simulink model "CAVE_MachE_speedTrack0202"  (R2019b)
settings: configuration reference "ConfigSetDesktopFixedStep" (kept outside this file)
PreLoadFcn:
  | VSS_BICYCLE=Simulink.Variant('Dual=0');
  | VSS_DUAL=Simulink.Variant('Dual=1');
  | Dual=1;
  | load('DriveCycle2.mat')
PostLoadFcn:
  | if any(exist('dsrtsu_mdlpostloadfcn', 'file') ~= 0), dsrtsu_mdlpostloadfcn('Execute', bdroot); end
InitFcn:
  | , if any(exist('dsmpb_private', 'file') ~= 0), dsmpb_private('dsmpb_mdlclblib', 'Init', bdroot); end,
  | load('DriveCycle2.mat')
model workspace (MAT data in the model file):
  Gas = 0.383333333333
values from neighbouring files (symbols this model uses):
  CoastDown =     [Run_Simulink.mat]
  limitedMCT =     [Run_Simulink.mat]
  MCT =     [Run_Simulink.mat]
  pMCT =     [Run_Simulink.mat]
  Ref_speed = [13 13.007895099 13.015778396 13.023649891 13.031509584 13.039357475 13.047193564 13.055017851 13.062830336 13.070631019 13.0784199 13.086196979 ... (2669 elements, 2669x1)]    [Ref_speed_and_time.mat]
  Ref_time = [0 0.01 0.02 0.03 0.04 0.05 0.06 0.07 0.08 0.09 0.1 0.11 ... (2669 elements, 2669x1)]    [Ref_speed_and_time.mat]
  US06 =     [Run_Simulink.mat]
undefined symbols (not defined in the file or in its folder): AccelCmd, ActTqLF_Nm_, ActTqLR_Nm_, ActTqRF_Nm_, ActTqRR_Nm_, BattChargeLimitMaxPwr, BattChargeLimitSocBpts, BattChargeLimitTbl, BattChrgCapcty, BattDischargeLimitSocBpts, BattDischargeLimitTbl, BattDischargeMaxPwr, BattNumCellsParallel, BattNumCellsSeries, BattOpenVoltCapBpts, BattOpenVoltTbl, BattResistSocBpts, BattResistTbl, BattResistTempBpts, BrakeMaxPrs, BrakeMaxTrq, ChassisDistCg2FrontAxle, ChassisDistCg2RearAxle, ChassisVehMass, CltchCmd, DecelCmd, DiffRatio, DiscIntNeverNeededParam, EnvGravCnst, EnvPrs, EnvTemp, FuelSpecificGrav, GearCmd, h, InitStates, lgSw, MtrEffSpdBpts, MtrEffTbl, MtrEffTrqBpts, MtrPwrMax, MtrTrqMax, Ref_Spd0229, Ref_Time0229, SteeringCmd, SupvsryCtrlRegenBrkCutOffTbl, SupvsryCtrlRegenSpdBpts, TestScnrioCycleNum, VEH
libraries: VSIGenLib x67, simulink x57, etargetslib x38, dsmpblib x28, vehdynlibtire x12, autolibshared x9, vehdynlibsuspension x7, vehdynlibtirecommon x7, autolibutils x5, CarMaker4SL x4, VsrLibWheel x4, autolibpowerinfoutils x3
(part 5 of 14)

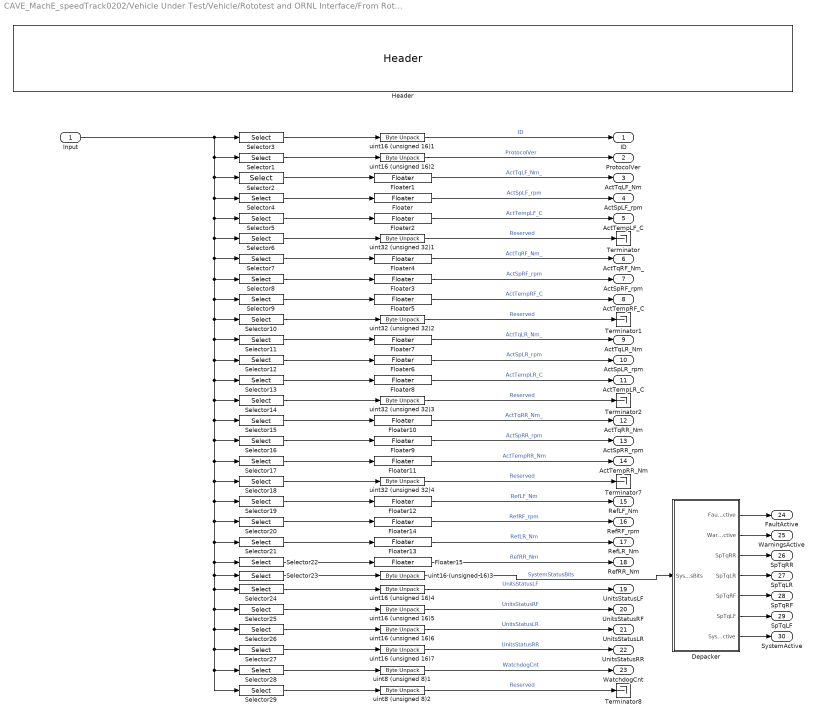
== system CAVE_MachE_speedTrack0202/Vehicle Under Test/Vehicle/Rototest and ORNL Interface/From Rototest/RotoTestEthRX ==
  Input : Inport
  Depacker : Subsystem
  Floater{,1..15} (16 alike) : VSIGenLib/Floater  SystemSampleTime=-1  Latency=0  AutoFrameSizeCalculation=off
  Header : VSIGenLib/Header  not=''
  Selector1 : Selector  IndexMode=Zero-based  InputPortWidth=96  IndexOptions=Index vector (dialog)  Indices=[3 2]  OutputSizes=1
  Selector10 : Selector  IndexMode=Zero-based  InputPortWidth=96  IndexOptions=Index vector (dialog)  Indices=[35 34 33 32]  OutputSizes=1
  Selector11 : Selector  IndexMode=Zero-based  InputPortWidth=96  IndexOptions=Index vector (dialog)  Indices=[39 38 37 36]  OutputSizes=1
  Selector12 : Selector  IndexMode=Zero-based  InputPortWidth=96  IndexOptions=Index vector (dialog)  Indices=[43 42 41 40]  OutputSizes=1
  Selector13 : Selector  IndexMode=Zero-based  InputPortWidth=96  IndexOptions=Index vector (dialog)  Indices=[47 46 45 44]  OutputSizes=1
  Selector14 : Selector  IndexMode=Zero-based  InputPortWidth=96  IndexOptions=Index vector (dialog)  Indices=[51 50 49 48]  OutputSizes=1
  Selector15 : Selector  IndexMode=Zero-based  InputPortWidth=96  IndexOptions=Index vector (dialog)  Indices=[55 54 53 52]  OutputSizes=1
  Selector16 : Selector  IndexMode=Zero-based  InputPortWidth=96  IndexOptions=Index vector (dialog)  Indices=[59 58 57 56]  OutputSizes=1
  Selector17 : Selector  IndexMode=Zero-based  InputPortWidth=96  IndexOptions=Index vector (dialog)  Indices=[63 62 61 60]  OutputSizes=1
  Selector18 : Selector  IndexMode=Zero-based  InputPortWidth=96  IndexOptions=Index vector (dialog)  Indices=[67 66 65 64]  OutputSizes=1
  Selector19 : Selector  IndexMode=Zero-based  InputPortWidth=96  IndexOptions=Index vector (dialog)  Indices=[71 70 69 68]  OutputSizes=1
  Selector2 : Selector  IndexMode=Zero-based  InputPortWidth=96  IndexOptions=Index vector (dialog)  Indices=[7 6 5 4]  OutputSizes=1
  Selector20 : Selector  IndexMode=Zero-based  InputPortWidth=96  IndexOptions=Index vector (dialog)  Indices=[75 74 73 72]  OutputSizes=1
  Selector21 : Selector  IndexMode=Zero-based  InputPortWidth=96  IndexOptions=Index vector (dialog)  Indices=[79 78 77 76]  OutputSizes=1
  Selector22 : Selector  IndexMode=Zero-based  InputPortWidth=96  IndexOptions=Index vector (dialog)  Indices=[83 82 81 80]  OutputSizes=1
  Selector23 : Selector  IndexMode=Zero-based  InputPortWidth=96  IndexOptions=Index vector (dialog)  Indices=[85 84]  OutputSizes=1
  Selector24 : Selector  IndexMode=Zero-based  InputPortWidth=96  IndexOptions=Index vector (dialog)  Indices=[87 86]  OutputSizes=1
  Selector25 : Selector  IndexMode=Zero-based  InputPortWidth=96  IndexOptions=Index vector (dialog)  Indices=[89 88]  OutputSizes=1
  Selector26 : Selector  IndexMode=Zero-based  InputPortWidth=96  IndexOptions=Index vector (dialog)  Indices=[91 90]  OutputSizes=1
  Selector27 : Selector  IndexMode=Zero-based  InputPortWidth=96  IndexOptions=Index vector (dialog)  Indices=[93 92]  OutputSizes=1
  Selector28 : Selector  IndexMode=Zero-based  InputPortWidth=96  IndexOptions=Index vector (dialog)  Indices=[94]  OutputSizes=1
  Selector29 : Selector  IndexMode=Zero-based  InputPortWidth=96  IndexOptions=Index vector (dialog)  Indices=[95]  OutputSizes=1
  Selector3 : Selector  IndexMode=Zero-based  InputPortWidth=96  IndexOptions=Index vector (dialog)  Indices=[1 0]  OutputSizes=1
  Selector4 : Selector  IndexMode=Zero-based  InputPortWidth=96  IndexOptions=Index vector (dialog)  Indices=[11 10 9 8]  OutputSizes=1
  Selector5 : Selector  IndexMode=Zero-based  InputPortWidth=96  IndexOptions=Index vector (dialog)  Indices=[15 14 13 12]  OutputSizes=1
  Selector6 : Selector  IndexMode=Zero-based  InputPortWidth=96  IndexOptions=Index vector (dialog)  Indices=[19 18 17 16]  OutputSizes=1
  Selector7 : Selector  IndexMode=Zero-based  InputPortWidth=96  IndexOptions=Index vector (dialog)  Indices=[23 22 21 20]  OutputSizes=1
  Selector8 : Selector  IndexMode=Zero-based  InputPortWidth=96  IndexOptions=Index vector (dialog)  Indices=[27 26 25 24]  OutputSizes=1
  Selector9 : Selector  IndexMode=Zero-based  InputPortWidth=96  IndexOptions=Index vector (dialog)  Indices=[31 30 29 28]  OutputSizes=1
  Terminator{,1..2,7..8} (5 alike) : Terminator
  uint16 (unsigned 16){1..7} (7 alike) : etargetslib/Byte Unpack  dimensions={[1]}  datatypes={'uint16'}  byteAlign=1
      settings: SourceProductName=MATLAB Coder
  uint32 (unsigned 32){1..4} (4 alike) : etargetslib/Byte Unpack  dimensions={[1]}  datatypes={'uint32'}  byteAlign=1
      settings: SourceProductName=MATLAB Coder
  uint8 (unsigned 8)1 : etargetslib/Byte Unpack  dimensions={[1]}  datatypes={'uint8'}  byteAlign=1
      settings: SourceProductName=MATLAB Coder
  uint8 (unsigned 8)2 : etargetslib/Byte Unpack  dimensions={[1]}  datatypes={'uint8'}  byteAlign=1
      settings: SourceProductName=MATLAB Coder
  ID : Outport
  ProtocolVer : Outport  Port=2
  ActTqLF_Nm : Outport  Port=3
  ActSpLF_rpm : Outport  Port=4
  ActTempLF_C : Outport  Port=5
  ActTqRF_Nm_ : Outport  Port=6
  ActSpRF_rpm : Outport  Port=7
  ActTempRF_C : Outport  Port=8
  ActTqLR_Nm : Outport  Port=9
  ActSpLR_rpm : Outport  Port=10
  ActTempLR_C : Outport  Port=11
  ActTqRR_Nm : Outport  Port=12
  ActSpRR_rpm : Outport  Port=13
  ActTempRR_Nm : Outport  Port=14
  RefLF_Nm : Outport  Port=15
  RefRF_rpm : Outport  Port=16
  RefLR_Nm : Outport  Port=17
  RefRR_Nm : Outport  Port=18
  UnitsStatusLF : Outport  Port=19
  UnitsStatusRF : Outport  Port=20
  UnitsStatusLR : Outport  Port=21
  UnitsStatusRR : Outport  Port=22
  WatchdogCnt : Outport  Port=23
  FaultActive : Outport  Port=24
  WarningsActive : Outport  Port=25
  SpTqRR : Outport  Port=26
  SpTqLR : Outport  Port=27
  SpTqRF : Outport  Port=28
  SpTqLF : Outport  Port=29
  SystemActive : Outport  Port=30
  wires:
  Depacker/7(SystemActive) -> SystemActive/1
  Depacker/5(SpTqRF) -> SpTqRF/1
  Depacker/1(FaultActive) -> FaultActive/1
  Depacker/2(WarningsActive) -> WarningsActive/1
  Depacker/3(SpTqRR) -> SpTqRR/1
  Depacker/4(SpTqLR) -> SpTqLR/1
  Depacker/6(SpTqLF) -> SpTqLF/1
  Floater5/1 -> ActTempRF_C/1  "ActTempRF_C"
  uint32 (unsigned 32)2/1 -> Terminator1/1  "Reserved"
  Floater/1 -> ActSpLF_rpm/1  "ActSpLF_rpm"
  uint32 (unsigned 32)1/1 -> Terminator/1  "Reserved"
  uint16 (unsigned 16)1/1 -> ID/1  "ID"
  Floater15/1 -> RefRR_Nm/1  "RefRR_Nm"
  uint8 (unsigned 8)1/1 -> WatchdogCnt/1  "WatchdogCnt"
  Floater14/1 -> RefRF_rpm/1  "RefRF_rpm"
  uint16 (unsigned 16)5/1 -> UnitsStatusRF/1  "UnitsStatusRF"
  uint32 (unsigned 32)3/1 -> Terminator2/1  "Reserved"
  Floater9/1 -> ActSpRR_rpm/1  "ActSpRR_rpm"
  Floater1/1 -> ActTqLF_Nm/1  "ActTqLF_Nm_"
  Floater2/1 -> ActTempLF_C/1  "ActTempLF_C"
  Floater12/1 -> RefLF_Nm/1  "RefLF_Nm"
  Floater7/1 -> ActTqLR_Nm/1  "ActTqLR_Nm_"
  uint16 (unsigned 16)2/1 -> ProtocolVer/1  "ProtocolVer"
  Selector24/1 -> uint16 (unsigned 16)4/1
  Selector7/1 -> Floater4/1
  Selector8/1 -> Floater3/1
  uint16 (unsigned 16)7/1 -> UnitsStatusRR/1  "UnitsStatusRR"
  Selector22/1 -> Floater15/1
  Selector18/1 -> uint32 (unsigned 32)4/1
  Selector12/1 -> Floater6/1
  Selector23/1 -> uint16 (unsigned 16)3/1
  uint16 (unsigned 16)6/1 -> UnitsStatusLR/1  "UnitsStatusLR"
  Selector17/1 -> Floater11/1
  uint16 (unsigned 16)4/1 -> UnitsStatusLF/1  "UnitsStatusLF"
  Selector27/1 -> uint16 (unsigned 16)7/1
  Floater13/1 -> RefLR_Nm/1  "RefLR_Nm"
  Selector14/1 -> uint32 (unsigned 32)3/1
  Selector2/1 -> Floater1/1
  Selector13/1 -> Floater8/1
  Selector26/1 -> uint16 (unsigned 16)6/1
  Selector6/1 -> uint32 (unsigned 32)1/1
  uint16 (unsigned 16)3/1 -> Depacker/1(SysStsBits)  "SystemStatusBits"
  uint32 (unsigned 32)4/1 -> Terminator7/1  "Reserved"
  Floater3/1 -> ActSpRF_rpm/1  "ActSpRF_rpm"
  Selector25/1 -> uint16 (unsigned 16)5/1
  Floater4/1 -> ActTqRF_Nm_/1  "ActTqRF_Nm_"
  uint8 (unsigned 8)2/1 -> Terminator8/1  "Reserved"
  Floater11/1 -> ActTempRR_Nm/1  "ActTempRR_Nm"
  Floater6/1 -> ActSpLR_rpm/1  "ActSpLR_rpm"
  Selector20/1 -> Floater14/1
  Selector9/1 -> Floater5/1
  Selector5/1 -> Floater2/1
  Selector15/1 -> Floater10/1
  Selector16/1 -> Floater9/1
  Floater8/1 -> ActTempLR_C/1  "ActTempLR_C"
  Selector3/1 -> uint16 (unsigned 16)1/1
  Selector28/1 -> uint8 (unsigned 8)1/1
  Selector29/1 -> uint8 (unsigned 8)2/1
  Selector21/1 -> Floater13/1
  Input/1 -> Selector7/1, Selector8/1, Selector9/1, Selector10/1, Selector11/1, Selector12/1, Selector13/1, Selector17/1, Selector18/1, Selector19/1, Selector20/1, Selector21/1, Selector22/1, Selector23/1, Selector25/1, Selector26/1, Selector27/1, Selector29/1, Selector28/1, Selector24/1, Selector16/1, Selector15/1, Selector14/1, Selector6/1, Selector5/1, Selector4/1, Selector2/1, Selector1/1, Selector3/1
  Selector19/1 -> Floater12/1
  Selector10/1 -> uint32 (unsigned 32)2/1
  Selector1/1 -> uint16 (unsigned 16)2/1
  Selector4/1 -> Floater/1
  Floater10/1 -> ActTqRR_Nm/1  "ActTqRR_Nm_"
  Selector11/1 -> Floater7/1

== system CAVE_MachE_speedTrack0202/Vehicle Under Test/Vehicle/Rototest and ORNL Interface/Get Wheel Spd Cmd Based on Wheel Dynamics/WheelSpdCmd ==
  In1 : Inport
  Bus Selector : BusSelector  OutputSignals=PT IF WFL rotv,PT IF WFR rotv,PT IF WRL rotv,PT IF WRR rotv
  Mux : Mux
  Out1 : Outport
  wires:
  Mux/1 -> Out1/1
  Bus Selector/1 -> Mux/1  "<PT IF WFL rotv>"
  Bus Selector/4 -> Mux/4  "<PT IF WRR rotv>"
  In1/1 -> Bus Selector/1
  Bus Selector/3 -> Mux/3  "<PT IF WRL rotv>"
  Bus Selector/2 -> Mux/2  "<PT IF WFR rotv>"

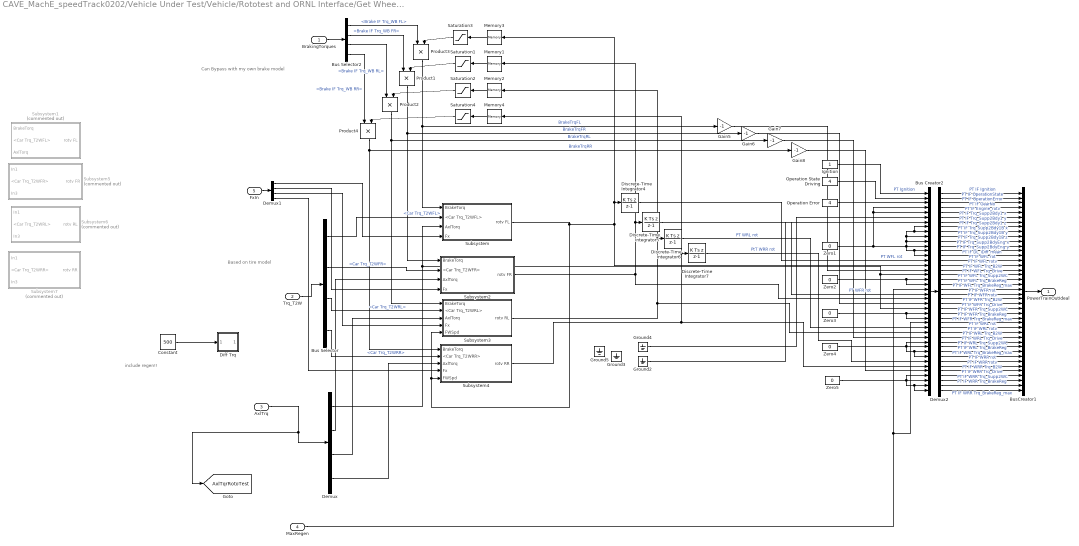
== system CAVE_MachE_speedTrack0202/Vehicle Under Test/Vehicle/Rototest and ORNL Interface/Get Wheel Spd Cmd Based on Wheel Dynamics/Whl Dynamics & Format CM Powertrain Signal ==
  note: include regen!!
  note: Based on tire model
  note: Can Bypass with my own brake model
  BrakingTorques : Inport
  Trq_T2W : Inport  Port=2
  AxlTrq : Inport  Port=3
  MaxRegen : Inport  Port=4
  FxIn : Inport  Port=5
  Bus Creator2 : BusCreator  Inputs=42
  Bus Selector : BusSelector  OutputSignals=Car Trq_T2WFL,Car Trq_T2WFR,Car Trq_T2WRL,Car Trq_T2WRR
  Bus Selector2 : BusSelector  OutputSignals=Brake IF Trq_WB FL,Brake IF Trq_WB FR,Brake IF Trq_WB RL,Brake IF Trq_WB RR
  BusCreator1 : BusCreator  Inputs=42
  Constant : Constant  Value=500
  Demux : Demux
  Demux1 : Demux
  Demux2 : Demux  Outputs=42
  Diff Trq : Subsystem
  Discrete-Time Integrator{4..7} (4 alike) : DiscreteIntegrator  IntegratorMethod=Integration: Backward Euler  SampleTime=-1  ICPrevOutput=DiscIntNeverNeededParam  ICPrevScaledInput=DiscIntNeverNeededParam
  Gain{5..8} (4 alike) : Gain  Gain=-1
  Ground{2..5} (4 alike) : Ground
  Ignition : Constant
  Memory{1..4} (4 alike) : Memory
  Operation Error : Constant  Value=4
  Operation State Driving : Constant  Value=4
  Product{1..4} (4 alike) : Product  RndMeth=Zero
  Saturation{1..4} (4 alike) : Saturate  UpperLimit=1  LowerLimit=-1
  Subsystem : Subsystem
  Subsystem1 : Subsystem  Commented=on
  Subsystem2 : Subsystem
  Subsystem3 : Subsystem
  Subsystem4 : Subsystem
  Subsystem5 : Subsystem  Commented=on
  Subsystem6 : Subsystem  Commented=on
  Subsystem7 : Subsystem  Commented=on
  Zero{1..5} (5 alike) : Constant  Value=0
  PowerTrainOutIdeal : Outport
  tag scope: AxlTqrRotoTest=global
  wires:
  Saturation4/1 -> Product4/2
  Memory4/1 -> Saturation4/1
  Bus Selector2/4 -> Product4/1  "<Brake IF Trq_WB RR>"
  Product4/1 -> Subsystem4/1(BrakeTorq), Gain8/1  "BrakeTrqRR"
  Saturation2/1 -> Product2/2
  Memory2/1 -> Saturation2/1
  Bus Selector2/3 -> Product2/1  "<Brake IF Trq_WB RL>"
  Product2/1 -> Subsystem3/1(BrakeTorq), Gain7/1  "BrakeTrqRL"
  Saturation1/1 -> Product1/2
  Memory1/1 -> Saturation1/1
  Bus Selector2/2 -> Product1/1  "<Brake IF Trq_WB FR>"
  Product1/1 -> Subsystem2/1(BrakeTorq), Gain6/1  "BrakeTrqFR"
  Memory3/1 -> Saturation3/1
  Saturation3/1 -> Product3/2
  Bus Selector2/1 -> Product3/1  "<Brake IF Trq_WB FL>"
  Product3/1 -> Subsystem/1(BrakeTorq), Gain5/1  "BrakeTrqFL"
  BrakingTorques/1 -> Bus Selector2/1
  Trq_T2W/1 -> Bus Selector/1
  Discrete-Time Integrator7/1 -> Bus Creator2/36  "PtT WRR rot"
  Discrete-Time Integrator6/1 -> Bus Creator2/29  "PT WRL rot"
  Discrete-Time Integrator5/1 -> Bus Creator2/22  "PT WFR rot"
  Discrete-Time Integrator4/1 -> Bus Creator2/15  "PT WFL rot"
  Ignition/1 -> Bus Creator2/1  "PT Ignition"
  Bus Creator2/1 -> Demux2/1
  Operation State Driving/1 -> Bus Creator2/2
  Operation Error/1 -> Bus Creator2/3
  Zero1/1 -> Bus Creator2/5, Bus Creator2/4, Bus Creator2/12, Bus Creator2/14, Bus Creator2/13, Bus Creator2/11, Bus Creator2/10, Bus Creator2/9, Bus Creator2/8
  Zero2/1 -> Bus Creator2/19, Bus Creator2/20
  Zero3/1 -> Bus Creator2/26, Bus Creator2/27
  Zero4/1 -> Bus Creator2/32, Bus Creator2/33, Bus Creator2/34, Bus Creator2/35
  Zero5/1 -> Bus Creator2/39, Bus Creator2/40, Bus Creator2/41, Bus Creator2/42
  Gain6/1 -> Bus Creator2/24
  Gain5/1 -> Bus Creator2/17
  Gain7/1 -> Bus Creator2/31
  Gain8/1 -> Bus Creator2/38
  Demux2/42 -> BusCreator1/42  "PT IF WRR Trq_BrakeReg_max"
  Demux2/41 -> BusCreator1/41  "PT IF WRR Trq_BrakeReg"
  Demux2/40 -> BusCreator1/40  "PT IF WRR Trq_Supp2WC"
  Demux2/39 -> BusCreator1/39  "PT IF WRR Trq_Drive"
  Demux2/38 -> BusCreator1/38  "PT IF WRR Trq_B2W"
  Demux2/37 -> BusCreator1/37  "PT IF WRR rotv"
  Demux2/36 -> BusCreator1/36  "PT IF WRR rot"
  Demux2/35 -> BusCreator1/35  "PT IF WRL Trq_BrakeReg_max"
  Demux2/34 -> BusCreator1/34  "PT IF WRL Trq_BrakeReg"
  Demux2/33 -> BusCreator1/33  "PT IF WRL Trq_Supp2WC"
  Demux2/32 -> BusCreator1/32  "PT IF WRL Trq_Drive"
  Demux2/31 -> BusCreator1/31  "PT IF WRL Trq_B2W"
  Demux2/30 -> BusCreator1/30  "PT IF WRL rotv"
  Demux2/29 -> BusCreator1/29  "PT IF WRL rot"
  Demux2/28 -> BusCreator1/28  "PT IF WFR Trq_BrakeReg_max"
  Demux2/27 -> BusCreator1/27  "PT IF WFR Trq_BrakeReg"
  Demux2/26 -> BusCreator1/26  "PT IF WFR Trq_Supp2WC"
  Demux2/25 -> BusCreator1/25  "PT IF WFR Trq_Drive"
  Demux2/24 -> BusCreator1/24  "PT IF WFR Trq_B2W"
  Demux2/23 -> BusCreator1/23  "PT IF WFR rotv"
  Demux2/22 -> BusCreator1/22  "PT IF WFR rot"
  Demux2/21 -> BusCreator1/21  "PT IF WFL Trq_BrakeReg_max"
  Demux2/20 -> BusCreator1/20  "PT IF WFL Trq_BrakeReg"
  Demux2/19 -> BusCreator1/19  "PT IF WFL Trq_Supp2WC"
  Demux2/18 -> BusCreator1/18  "PT IF WFL Trq_Drive"
  Demux2/17 -> BusCreator1/17  "PT IF WFL Trq_B2W"
  Demux2/16 -> BusCreator1/16  "PT IF WFL rotv"
  Demux2/15 -> BusCreator1/15  "PT IF WFL rot"
  Demux2/14 -> BusCreator1/14  "PT IF DL_iDiff_mean"
  Demux2/13 -> BusCreator1/13  "PT IF Trq_Supp2BdyEng y"
  Demux2/12 -> BusCreator1/12  "PT IF Trq_Supp2BdyEng x"
  Demux2/11 -> BusCreator1/11  "PT IF Trq_Supp2Bdy1B z"
  Demux2/10 -> BusCreator1/10  "PT IF Trq_Supp2Bdy1B y"
  Demux2/9 -> BusCreator1/9  "PT IF Trq_Supp2Bdy1B x"
  Demux2/8 -> BusCreator1/8  "PT IF Trq_Supp2Bdy1 z"
  Demux2/7 -> BusCreator1/7  "PT IF Trq_Supp2Bdy1 y"
  Demux2/6 -> BusCreator1/6  "PT IF Trq_Supp2Bdy1 x"
  Demux2/5 -> BusCreator1/5  "PT IF Engine_rotv"
  Demux2/4 -> BusCreator1/4  "PT IF GearNo"
  Demux2/3 -> BusCreator1/3  "PT IF OperationError"
  Demux2/2 -> BusCreator1/2  "PT IF OperationState"
  Demux2/1 -> BusCreator1/1  "PT IF Ignition"
  BusCreator1/1 -> PowerTrainOutIdeal/1
  Ground2/1 -> Bus Creator2/7
  Ground4/1 -> Bus Creator2/6
  Constant/1 -> Diff Trq/1(In1)
  AxlTrq/1 -> [AxlTqrRotoTest], Demux/1
  Demux/1 -> Subsystem/3(AxlTorq), Bus Creator2/25, Bus Creator2/18
  MaxRegen/1 -> Bus Creator2/28, Bus Creator2/21
  Subsystem/1(rotv FL) -> Subsystem3/5(FWSpd), Subsystem4/5(FWSpd), Bus Creator2/16, Memory3/1, Discrete-Time Integrator4/1
  Bus Selector/1 -> Subsystem/2(<Car Trq_T2WFL>)  "<Car Trq_T2WFL>"
  Subsystem2/1(rotv FR) -> Bus Creator2/23, Memory1/1, Discrete-Time Integrator5/1
  Bus Selector/2 -> Subsystem2/2(<Car Trq_T2WFR>)  "<Car Trq_T2WFR>"
  Demux/2 -> Subsystem2/3(AxlTorq)
  Subsystem3/1(rotv RL) -> Memory2/1, Discrete-Time Integrator6/1, Bus Creator2/30
  Bus Selector/3 -> Subsystem3/2(<Car Trq_T2WRL>)  "<Car Trq_T2WRL>"
  Demux/3 -> Subsystem3/3(AxlTorq)
  Subsystem4/1(rotv RR) -> Memory4/1, Discrete-Time Integrator7/1, Bus Creator2/37
  Bus Selector/4 -> Subsystem4/2(<Car Trq_T2WRR>)  "<Car Trq_T2WRR>"
  Demux/4 -> Subsystem4/3(AxlTorq)
  FxIn/1 -> Demux1/1
  Demux1/1 -> Subsystem/4(Fx)
  Demux1/2 -> Subsystem2/4(Fx)
  Demux1/3 -> Subsystem3/4(Fx)
  Demux1/4 -> Subsystem4/4(Fx)

== system CAVE_MachE_speedTrack0202/Vehicle Under Test/Vehicle/Rototest and ORNL Interface/To Rototest with Band-Aid/Band-Aid ==
  InSpd_rpm : Inport
  InTrq_Nm : Inport  Port=2
  BRAKE_PRESSED : Inport  Port=3
  VehSpd_kph : Inport  Port=4
  Band-Aid : Stateflow chart  BlockKeywords=__PRM__SERIALIZED__DATA__:Stateflow Chart,Stateflow Diagram  TreatAsAtomicUnit=on
  BrkLatchThr_Nm : Constant  Value=-50
  Header : VSIGenLib/Header  not=''
  LaunchSpdThr_rpm : Constant  Value=2
  LaunchTrqThr_Nm : Constant  Value=20
  SettleTime_s : Constant  Value=5
  SpdLatchThr_rpm : Constant  Value=1e-5
  Terminator : Terminator
  Terminator1 : Terminator
  VehSpdThr_kph : Constant  Value=0.2
  dStop : Constant  Value=0
  OutMode : Outport
  OutSpd_rpm : Outport  Port=2
  tag scope: Mode=global
  wires:
  InSpd_rpm/1 -> Band-Aid/5(InSpd)  "InSpd_rpm"
  LaunchTrqThr_Nm/1 -> Band-Aid/2(LaunchTrqThr)
  SpdLatchThr_rpm/1 -> Band-Aid/3(SpdLatchThr)
  Band-Aid/3(State) -> Terminator/1  "State"
  LaunchSpdThr_rpm/1 -> Band-Aid/1(LaunchSpdThr)
  SettleTime_s/1 -> Band-Aid/7(SettleTime)
  Band-Aid/1(OutMode) -> [Mode], OutMode/1  "OutMode"
  BrkLatchThr_Nm/1 -> Terminator1/1
  Band-Aid/2(OutSpd) -> OutSpd_rpm/1  "OutSpd"
  InTrq_Nm/1 -> Band-Aid/6(InTrq)  "InTrq_Nm"
  dStop/1 -> Band-Aid/8(dStop)
  BRAKE_PRESSED/1 -> Band-Aid/4(BrkSw)
  VehSpd_kph/1 -> Band-Aid/9(VehSpd_kph)  "VehicleSpeed_kph"
  VehSpdThr_kph/1 -> Band-Aid/10(VehSpdThr_kph)

== system CAVE_MachE_speedTrack0202/Vehicle Under Test/Vehicle/Rototest and ORNL Interface/To Rototest with Band-Aid/Logging ==
  Ground1 : Ground
  RotoTestEthRXLogging : Subsystem
      mask Display:
      | color('white')
      | disp('RotTestEthLog')
      | port_label('output', 1, 'ID')
      | port_label('output', 2, 'ProtocolVer')
      | port_label('output', 3, 'ActTqLF (Nm)')
      | port_label('output', 4, 'ActSpdLF (rpm)')
      | port_label('output', 5, 'ActTempLF (C)')
      | port_label('output', 6, 'ActTqRF (Nm)')
      | port_label('output', 7, 'ActSpRF (rpm)')
      | port_label('output', 8, 'ActTempRF (C)')
      | port_label('output', 9, 'ActTqLR (Nm)')
      | port_label('output', 10, 'ActSpLR (rpm)')
      | port_label('output', 11, 'ActTempLR (C)')
      | port_label('output', 12, 'ActTqRR (Nm)')
      | port_label('output', 13, 'ActSpRR (rpm)')
      | port_label('output', 14, 'ActTempRR (Nm)')
      | port_label('output', 15, 'ActTqDeltaF (Nm)')
      | port_label('output', 16, 'ActSpDeltaF (rpm)')
      | port_label('output', 17, 'ActTqDeltaR (Nm)')
      | port_label('output', 18, 'ActSpDeltaR (rpm)')
      | port_label('output', 19, 'ActTqDeltaA (Nm')
      | port_label('output', 20, 'ActSqDeltaA (rpm)')
      | port_label('output', 21, 'ActTqTot (Nm)')
      | port_label('output', 22, 'ActSpAve (rpm)')
      | port_label('output', 23, 'ActPow (kW)')
      | port_label('output', 24, 'ActVehSp (kph)')
      | port_label('output', 25, 'TPTime (ms)')
      | port_label('output', 26, 'TPDistance (m)')
      | port_label('output', 27, 'FaultActive (bool)')
      | port_label('output', 28, 'WarningsActive (bool)')
      | port_label('output', 29, 'MeasuringStatus (bool)')
      | port_label('output', 30, 'SystemActive (bool)')
      | 
      | port_label('output', 31, 'UnitStatusLF (enum)')
      | port_label('output', 32, 'UnitStatusRF (enum)')
      | port_label('output', 33, 'UnitStatusLR (enum)')
      | port_label('output', 34, 'UnitStatusRR (enum)')
      | port_label('output', 35, 'WatchdogCnt (int)')
  Terminator{28..62} (35 alike) : Terminator
  wires:
  RotoTestEthRXLogging/24(ActVehSp_kph) -> Terminator51/1
  RotoTestEthRXLogging/9(ActTqLR_Nm) -> Terminator30/1
  RotoTestEthRXLogging/11(ActTempLR_C) -> Terminator38/1
  RotoTestEthRXLogging/5(ActTempLF_C) -> Terminator28/1
  RotoTestEthRXLogging/12(ActTqRR_Nm) -> Terminator39/1
  RotoTestEthRXLogging/10(ActSpLR_rpm) -> Terminator31/1
  RotoTestEthRXLogging/8(ActTempRF_C) -> Terminator33/1
  RotoTestEthRXLogging/26(TPDistance_m) -> Terminator59/1
  RotoTestEthRXLogging/19(ActTqDeltaA_Nm) -> Terminator44/1
  RotoTestEthRXLogging/6(ActTqRF_Nm) -> Terminator29/1
  RotoTestEthRXLogging/4(ActSpLF_rpm) -> Terminator37/1
  RotoTestEthRXLogging/1(ID) -> Terminator34/1
  RotoTestEthRXLogging/14(ActTempRR_Nm) -> Terminator47/1
  RotoTestEthRXLogging/30(SystemActive) -> Terminator53/1
  RotoTestEthRXLogging/22(ActSpAve_rpm) -> Terminator43/1
  RotoTestEthRXLogging/13(ActSpRR_rpm) -> Terminator46/1
  RotoTestEthRXLogging/31(UnitsStatusLF) -> Terminator56/1
  RotoTestEthRXLogging/21(ActTqTot_Nm) -> Terminator42/1
  RotoTestEthRXLogging/17(ActTqDeltaR_Nm) -> Terminator40/1
  RotoTestEthRXLogging/7(ActSpRF_rpm) -> Terminator32/1
  RotoTestEthRXLogging/2(ProtocolVer) -> Terminator35/1
  RotoTestEthRXLogging/16(ActSpDeltaF_rpm) -> Terminator49/1
  RotoTestEthRXLogging/18(ActSpDeltaR_rpm) -> Terminator41/1
  RotoTestEthRXLogging/15(ActTqDeltaF_Nm) -> Terminator48/1
  RotoTestEthRXLogging/33(UnitsStatusLR) -> Terminator54/1
  RotoTestEthRXLogging/23(ActPow_kW) -> Terminator50/1
  RotoTestEthRXLogging/25(TPTime_ms) -> Terminator58/1
  RotoTestEthRXLogging/28(WarningsActive) -> Terminator61/1
  RotoTestEthRXLogging/27(FaultActive) -> Terminator60/1
  RotoTestEthRXLogging/35(WatchdogCnt) -> Terminator62/1
  RotoTestEthRXLogging/34(UnitsStatusRR) -> Terminator55/1
  RotoTestEthRXLogging/20(ActSpDeltaA_rpm) -> Terminator45/1
  RotoTestEthRXLogging/32(UnitsStatusRF) -> Terminator57/1
  RotoTestEthRXLogging/29(MeasuringStatus) -> Terminator52/1
  RotoTestEthRXLogging/3(ActTqLF_Nm) -> Terminator36/1
  Ground1/1 -> RotoTestEthRXLogging/1(Cmd)

== system CAVE_MachE_speedTrack0202/Vehicle Under Test/Vehicle/Rototest and ORNL Interface/To Rototest with Band-Aid/Mode Override ==
  Header : VSIGenLib/Header  not=''
  Mux6 : Mux
  SpTqLF : Constant  Value=0  OutDataTypeStr=uint8
  SpTqLR : Constant  Value=0  OutDataTypeStr=uint8
  SpTqRF : Constant  Value=0  OutDataTypeStr=uint8
  SpTqRR : Constant  Value=0  OutDataTypeStr=uint8
  Ovr : Outport
  wires:
  Mux6/1 -> Ovr/1
  SpTqRR/1 -> Mux6/1
  SpTqLR/1 -> Mux6/2
  SpTqRF/1 -> Mux6/3
  SpTqLF/1 -> Mux6/4

== system CAVE_MachE_speedTrack0202/Vehicle Under Test/Vehicle/Rototest and ORNL Interface/To Rototest with Band-Aid/RotoTestEthTx ==
  RefLF_NmORrpm : Inport
  RefRF_NmORrpm : Inport  Port=2
  RefLR_NmORrpm : Inport  Port=3
  RefRR_NmORrpm : Inport  Port=4
  SpTqRR : Inport  Port=5
  SpTqLR : Inport  Port=6
  SpTqRF : Inport  Port=7
  SpTqLF : Inport  Port=8
  SystemActive : Inport  Port=9
  Constant : Constant  Value=255  OutDataTypeStr=uint8
  Constant1 : Constant  Value=0  OutDataTypeStr=uint8
  Constant2 : Constant  Value=0  OutDataTypeStr=uint8
  Constant3 : Constant  Value=0  OutDataTypeStr=uint8
  Defloater{,1..3} (4 alike) : VSIGenLib/Defloater  SystemSampleTime=-1  Latency=0  AutoFrameSizeCalculation=off
  Demux{,1..3} (4 alike) : Demux
  Header : VSIGenLib/Header  not=''
  ID1 : Constant  Value=hex2dec('D3')  OutDataTypeStr=uint8
  ID2 : Constant  Value=hex2dec('02')  OutDataTypeStr=uint8
  MATLAB Function : MATLAB Function  TreatAsAtomicUnit=on
  Mux : Mux  Inputs=25
  Packer : Subsystem
  ProtocolVer : Constant  Value=0  OutDataTypeStr=uint16
  SystemCtrlBits2 : Constant  Value=0  OutDataTypeStr=uint8
  Terminator : Terminator
  WatchdogCnt : simulink/Sources/Counter Free-Running  NumBits=8  tsamp=-1
  uint16 (unsigned 16) 2 : etargetslib/Byte Pack  datatypes={'uint16'}  byteAlign=1
      settings: SourceProductName=MATLAB Coder
  uint8 (unsigned 8) {1..9} (9 alike) : etargetslib/Byte Pack  datatypes={'uint8'}  byteAlign=1
      settings: SourceProductName=MATLAB Coder
  Output : Outport
  wires:
  Defloater2/1 -> Demux2/1
  ID2/1 -> uint8 (unsigned 8) 7/1
  RefRF_NmORrpm/1 -> Defloater1/1  "RefRF_NmORrpm"
  Demux1/4 -> Mux/11
  Constant1/1 -> uint8 (unsigned 8) 4/1  "Reserved25"
  WatchdogCnt/1 -> uint8 (unsigned 8) 1/1  "WatchdogCnt"
  Defloater3/1 -> Demux3/1
  Demux3/3 -> Mux/18
  uint8 (unsigned 8) 5/1 -> Mux/21
  Demux1/3 -> Mux/10
  uint8 (unsigned 8) 2/1 -> Mux/23
  Constant2/1 -> uint8 (unsigned 8) 3/1  "Reserved24"
  ID1/1 -> uint8 (unsigned 8) 8/1
  uint8 (unsigned 8) 4/1 -> Mux/25
  Demux/1 -> Mux/4
  Demux3/1 -> Mux/16
  Demux1/1 -> Mux/8
  ProtocolVer/1 -> uint16 (unsigned 16) 2/1
  uint8 (unsigned 8) 3/1 -> Mux/24
  Demux2/2 -> Mux/13
  uint8 (unsigned 8) 1/1 -> Mux/22
  uint16 (unsigned 16) 2/1 -> Mux/3
  Defloater1/1 -> Demux1/1
  Defloater/1 -> Demux/1
  Demux2/1 -> Mux/12
  Demux/4 -> Mux/7
  Demux2/3 -> Mux/14
  MATLAB Function/1(y) -> uint8 (unsigned 8) 9/1  "Ref_Byte"
  Demux1/2 -> Mux/9
  Demux/3 -> Mux/6
  Mux/1 -> Output/1  "bytesend"
  uint8 (unsigned 8) 8/1 -> Mux/1
  Demux2/4 -> Mux/15
  Demux3/4 -> Mux/19
  SystemCtrlBits2/1 -> uint8 (unsigned 8) 5/1  "SystemCtrlBits2"
  uint8 (unsigned 8) 7/1 -> Mux/2
  RefRR_NmORrpm/1 -> Defloater3/1  "RefRR_NmORrpm"
  Demux/2 -> Mux/5
  Constant3/1 -> uint8 (unsigned 8) 2/1  "Reserved23"
  Demux3/2 -> Mux/17
  RefLF_NmORrpm/1 -> Defloater/1  "RefLF_NmORrpm"
  RefLR_NmORrpm/1 -> Defloater2/1  "RefLR_NmORrpm"
  SpTqRR/1 -> MATLAB Function/1(SpTqRR), Packer/1(SpTqRR)  "SpTqRR"
  SpTqLR/1 -> MATLAB Function/2(SpTqLR), Packer/2(SpTqLR)  "SpTqLR"
  SpTqRF/1 -> MATLAB Function/3(SpTqRF), Packer/3(SpTqRF)  "SpTqRF"
  SpTqLF/1 -> MATLAB Function/4(SpTqLF), Packer/4(SpTqLF)  "SpTqLF"
  SystemActive/1 -> MATLAB Function/5(SystemActive), Packer/5(SystemActive)
  Packer/1(SystemCtrlBits) -> Terminator/1
  Constant/1 -> uint8 (unsigned 8) 6/1
  uint8 (unsigned 8) 9/1 -> Mux/20

== system CAVE_MachE_speedTrack0202/Vehicle Under Test/Vehicle/Rototest and ORNL Interface/To Rototest with Band-Aid/TrqSpd Override ==
  Header : VSIGenLib/Header  not=''
  Mux2 : Mux
  RefLF_NmORrpm : Constant  Value=0
  RefLR_NmORrpm : Constant  Value=0
  RefRF_NmORrpm : Constant  Value=0
  RefRR_NmORrpm : Constant  Value=0
  Ovr : Outport
  wires:
  RefRF_NmORrpm/1 -> Mux2/2
  RefLF_NmORrpm/1 -> Mux2/1
  RefLR_NmORrpm/1 -> Mux2/3
  RefRR_NmORrpm/1 -> Mux2/4
  Mux2/1 -> Ovr/1

== system CAVE_MachE_speedTrack0202/Vehicle Under Test/Vehicle/Vehicle Dynamics/Vehicle 14DOF/Brake Pressure ==
  BrkReq : Inport
  Bus Creator1 : BusCreator  Inputs=2
  Gain : Gain  Gain=BrakeMaxPrs
  Gain{1..4} (4 alike) : Gain  Gain=0.5
  Saturation{,1..3} (4 alike) : Saturate  UpperLimit=BrakeMaxPrs  LowerLimit=0  ZeroCross=off
  Signal Specification : SignalSpecification  Unit=Pa
  Terminator : Terminator
  Vector Concatenate2 : Concatenate  NumInputs=4
  BrakePrs : Outport  Unit=Pa
  wires:
  BrkReq/1 -> Gain/1, Bus Creator1/1  "BrkReq"
  Gain/1 -> Signal Specification/1
  Signal Specification/1 -> Gain2/1, Gain1/1, Bus Creator1/2  "BrkPrs"
  Bus Creator1/1 -> Terminator/1  "WhlBrk"
  Gain1/1 -> Gain4/1
  Gain2/1 -> Gain3/1
  Gain3/1 -> Saturation/1, Saturation1/1
  Gain4/1 -> Saturation2/1, Saturation3/1
  Vector Concatenate2/1 -> BrakePrs/1
  Saturation/1 -> Vector Concatenate2/1
  Saturation1/1 -> Vector Concatenate2/2
  Saturation2/1 -> Vector Concatenate2/3
  Saturation3/1 -> Vector Concatenate2/4

== system CAVE_MachE_speedTrack0202/Vehicle Under Test/Vehicle/Vehicle Dynamics/Vehicle 14DOF/Steering ==
  SteeringCmd : Inport
  Constant : Constant  Value=0
  Kinematic Steering : vehdynlibsteering/Kinematic Steering  StrgType=Parallel  StrgRatioType=Constant  Loc=Front  NrmlFctr=1  TrckWdth=1.9  WhlBase=ChassisDistCg2FrontAxle+ChassisDistCg2RearAxle  Db=0  StrgRng=2.91*pi  StrgAngBpts="[-6.2832   -5.0265   -3.7699   -2.5133   -1.2566         0    1.2566    2.5133    3.7699    5.0265    6.2832]"  StrgRatioTbl=|  StrgRatio=16.8  StrgArmLngth=0.1  RckCsLngth=0.5  TieRodLngth=0.248  D=0.2  PnnRadius=0.0057  PnnRadiusTbl="[0.0055    0.0055    0.0056    0.0057    0.0058    0.0057    0.0057    0.0057    0.0056    0.0055    0.0055]"  RodLngth=0.1  ParaArmLngth=0.9  aMode=2
      | [13.5000   13.3750   13.2500   13.1250   13.0000   13.0000   13.0000   13.1250   13.2500   13.3750   13.5000
      | ]
      settings: SourceProductName=Vehicle Dynamics Blockset
  Terminator1 : Terminator
  Vector Concatenate : Concatenate
  Vector Concatenate1 : Concatenate
  Vector Concatenate2 : Concatenate
  WhlAng : Outport  Unit=rad
  wires:
  Kinematic Steering/1 -> Terminator1/1
  Vector Concatenate2/1 -> WhlAng/1
  Kinematic Steering/2 -> Vector Concatenate/1
  Vector Concatenate1/1 -> Vector Concatenate2/2  "RearWheelAngles"
  Vector Concatenate/1 -> Vector Concatenate2/1  "FrontWheelAngles"
  Constant/1 -> Vector Concatenate1/2, Vector Concatenate1/1
  Kinematic Steering/3 -> Vector Concatenate/2
  SteeringCmd/1 -> Kinematic Steering/1

== system CAVE_MachE_speedTrack0202/Vehicle Under Test/Vehicle/Vehicle Dynamics/Vehicle 14DOF/Subsystem4 ==
  Cgxyzdot : Inport
  CgXYZ : Inport  Port=2
  CgXYZdot : Inport  Port=3
  angles : Inport  Port=4
  pqr : Inport  Port=5
  Cgaxyz : Inport  Port=6
  Beta : Inport  Port=7
  GeomXYZ : Inport  Port=8
  GeomXYZdot : Inport  Port=9
  Omega : Inport  Port=10
  Kappa : Inport  Port=11
  Alpha : Inport  Port=12
  XWheel : Inport  Port=13
  YWheel : Inport  Port=14
  dzWheel : Inport  Port=15
  Bus Creator : BusCreator  Inputs=26
  Bus Creator3 : BusCreator  Inputs=6
  Demux{,1..7} (8 alike) : Demux  Outputs=3
  Subsystem : Subsystem
  Chassis : Outport  VectorParamsAs1DForOutWhenUnconnected=off
  Wheels : Outport  Port=2  VectorParamsAs1DForOutWhenUnconnected=off
  wires:
  Bus Creator/1 -> Chassis/1  "Chassis"
  Omega/1 -> Bus Creator3/3  "Omega"
  dzWheel/1 -> Bus Creator3/6  "dZWheel"
  Kappa/1 -> Bus Creator3/1  "Kappa"
  Bus Creator3/1 -> Wheels/1  "Wheels"
  YWheel/1 -> Bus Creator3/5  "YWheel"
  XWheel/1 -> Bus Creator3/4  "XWheel"
  Alpha/1 -> Bus Creator3/2  "Alpha"
  Cgxyzdot/1 -> Subsystem/1(Cgxyzdot), Demux/1
  CgXYZ/1 -> Demux1/1
  CgXYZdot/1 -> Demux2/1
  angles/1 -> Subsystem/2(angles), Demux3/1
  pqr/1 -> Demux4/1
  Cgaxyz/1 -> Demux5/1
  GeomXYZdot/1 -> Demux7/1
  GeomXYZ/1 -> Demux6/1
  Demux/1 -> Bus Creator/1  "xdot"
  Demux/2 -> Bus Creator/2  "ydot"
  Demux/3 -> Bus Creator/3  "zdot"
  Demux1/1 -> Bus Creator/4  "X"
  Demux1/2 -> Bus Creator/5  "Y"
  Demux1/3 -> Bus Creator/6  "Z"
  Demux2/1 -> Bus Creator/7  "Xdot"
  Demux2/2 -> Bus Creator/8  "Ydot"
  Demux2/3 -> Bus Creator/9  "Zdot"
  Demux3/1 -> Bus Creator/10  "phi"
  Demux3/2 -> Bus Creator/11  "theta"
  Demux3/3 -> Bus Creator/12  "psi"
  Demux4/1 -> Bus Creator/13  "p"
  Demux4/2 -> Bus Creator/14  "q"
  Demux4/3 -> Bus Creator/15  "r"
  Demux5/1 -> Bus Creator/16  "ax"
  Demux5/2 -> Bus Creator/17  "ay"
  Demux5/3 -> Bus Creator/18  "az"
  Beta/1 -> Bus Creator/19  "Beta"
  Demux6/1 -> Bus Creator/20  "GeomX"
  Demux6/2 -> Bus Creator/21  "GeomY"
  Demux6/3 -> Bus Creator/22  "GeomZ"
  Demux7/1 -> Bus Creator/23  "GeomXdot"
  Demux7/2 -> Bus Creator/24  "GeomYdot"
  Demux7/3 -> Bus Creator/25  "GeomZdot"
  Subsystem/1(VehSpd) -> Bus Creator/26  "VehSpd"

== system CAVE_MachE_speedTrack0202/Vehicle Under Test/Vehicle/Vehicle Dynamics/Vehicle 14DOF/Suspension ==
  Steering : Inport
  Vehicle : Inport  Port=2
  Wheel : Inport  Port=3
  Double Wishbone Suspension : Subsystem  VariantControl=1
      mask Display: image('suspdw.png');
  Independent Mapped Front Suspension Mapped Solid Axle Rear Suspension : Subsystem  VariantControl=2
      mask Display: image([imread('suspindmap.png');imread('suspsamap.png')]);
  MacPherson Front Suspension Solid Axle Rear Suspension : Subsystem  VariantControl=3
      mask Display: image([imread('suspmacp.png');imread('suspsacoil.png')]);
  MacPherson Suspension : Subsystem  VariantControl=4
      mask Display: image('suspmacp.png');
  Mapped Suspension : Subsystem  VariantControl=5
      mask Display: image('suspindmap.png');
  Suspension : Outport  VectorParamsAs1DForOutWhenUnconnected=off

== system CAVE_MachE_speedTrack0202/Vehicle Under Test/Vehicle/Vehicle Dynamics/Vehicle 14DOF/Vehicle ==
  Suspension : Inport
  Wind : Inport  Port=2
  Variant Subsystem : Subsystem  VariantControlMode=Label  Variant=on  LabelModeActiveChoice=1
  VehFdbk : Outport  VectorParamsAs1DForOutWhenUnconnected=off
  wires:
  Variant Subsystem/1(VehFdbk) -> VehFdbk/1  "VehFdbk"
  Wind/1 -> Variant Subsystem/2(Wind)
  Suspension/1 -> Variant Subsystem/1(Suspension)

== system CAVE_MachE_speedTrack0202/Vehicle Under Test/Vehicle/Vehicle Dynamics/Vehicle 14DOF/Vehicle Routing ==
  Veh : Inport
  Bus Selector10 : BusSelector  OutputSignals=BdyFrm.Cg.Vel.xdot,BdyFrm.Cg.Vel.ydot,BdyFrm.Cg.Vel.zdot  OutputAsBus=on
  Bus Selector2 : BusSelector  OutputSignals=InertFrm.Cg.Disp.X,InertFrm.Cg.Disp.Y,InertFrm.Cg.Disp.Z  OutputAsBus=on
  Bus Selector3 : BusSelector  OutputSignals=InertFrm.Cg.Vel.Xdot,InertFrm.Cg.Vel.Ydot,InertFrm.Cg.Vel.Zdot  OutputAsBus=on
  Bus Selector4 : BusSelector  OutputSignals=BdyFrm.Cg.Acc.ax,BdyFrm.Cg.Acc.ay,BdyFrm.Cg.Acc.az  OutputAsBus=on
  Bus Selector5 : BusSelector  OutputSignals=InertFrm.Cg.Ang.phi,InertFrm.Cg.Ang.theta,InertFrm.Cg.Ang.psi  OutputAsBus=on
  Bus Selector6 : BusSelector  OutputSignals=BdyFrm.Cg.AngVel.p,BdyFrm.Cg.AngVel.q,BdyFrm.Cg.AngVel.r  OutputAsBus=on
  Bus Selector7 : BusSelector  OutputSignals=InertFrm.Geom.Disp.X,InertFrm.Geom.Disp.Y,InertFrm.Geom.Disp.Z  OutputAsBus=on
  Bus Selector8 : BusSelector  OutputSignals=InertFrm.Geom.Vel.Xdot,InertFrm.Geom.Vel.Ydot,InertFrm.Geom.Vel.Zdot  OutputAsBus=on
  Bus Selector9 : BusSelector  OutputSignals=BdyFrm.Geom.Ang.Beta
  Bus to Vector{1..8} (8 alike) : BusToVector
  Cgxyzdot : Outport  VectorParamsAs1DForOutWhenUnconnected=off
  CgXYZ : Outport  Port=2  VectorParamsAs1DForOutWhenUnconnected=off
  CgXYZdot : Outport  Port=3  VectorParamsAs1DForOutWhenUnconnected=off
  angles : Outport  Port=4  VectorParamsAs1DForOutWhenUnconnected=off
  pqr : Outport  Port=5  VectorParamsAs1DForOutWhenUnconnected=off
  Cgaxyz : Outport  Port=6  VectorParamsAs1DForOutWhenUnconnected=off
  Beta : Outport  Port=7  VectorParamsAs1DForOutWhenUnconnected=off
  GeomXYZ : Outport  Port=8  VectorParamsAs1DForOutWhenUnconnected=off
  GeomXYZdot : Outport  Port=9  VectorParamsAs1DForOutWhenUnconnected=off
  wires:
  Bus Selector3/1 -> Bus to Vector2/1
  Bus to Vector1/1 -> CgXYZ/1
  Bus to Vector5/1 -> pqr/1
  Bus Selector5/1 -> Bus to Vector4/1
  Bus Selector6/1 -> Bus to Vector5/1
  Bus to Vector4/1 -> angles/1
  Bus to Vector8/1 -> Cgxyzdot/1
  Bus Selector2/1 -> Bus to Vector1/1
  Bus Selector8/1 -> Bus to Vector7/1
  Bus to Vector6/1 -> GeomXYZ/1
  Bus Selector9/1 -> Beta/1  "<Beta>"
  Bus Selector4/1 -> Bus to Vector3/1
  Bus Selector10/1 -> Bus to Vector8/1
  Bus to Vector7/1 -> GeomXYZdot/1
  Bus to Vector3/1 -> Cgaxyz/1
  Bus Selector7/1 -> Bus to Vector6/1
  Bus to Vector2/1 -> CgXYZdot/1
  Veh/1 -> Bus Selector8/1, Bus Selector7/1, Bus Selector9/1, Bus Selector4/1, Bus Selector6/1, Bus Selector5/1, Bus Selector3/1, Bus Selector2/1, Bus Selector10/1

== system CAVE_MachE_speedTrack0202/Vehicle Under Test/Vehicle/Vehicle Dynamics/Vehicle 14DOF/Wheel Routing ==
  Info : Inport
  Wheel : Inport  Port=2
  Bus Selector : BusSelector  OutputSignals=InertFrm.FrntAxl.Lft.Disp.Y,InertFrm.FrntAxl.Rght.Disp.Y,InertFrm.RearAxl.Lft.Disp.Y,InertFrm.RearAxl.Rght.Disp.Y
  Bus Selector1 : BusSelector  OutputSignals=InertFrm.FrntAxl.Lft.Disp.X,InertFrm.FrntAxl.Rght.Disp.X,InertFrm.RearAxl.Lft.Disp.X,InertFrm.RearAxl.Rght.Disp.X
  Bus Selector2 : BusSelector  OutputSignals=TireFrame.z,TireFrame.Omega,TireFrame.Kappa,TireFrame.Alpha
  Bus Selector3 : BusSelector  OutputSignals=InertFrm.FrntAxl.Lft.Disp.Z,InertFrm.FrntAxl.Rght.Disp.Z,InertFrm.RearAxl.Lft.Disp.Z,InertFrm.RearAxl.Rght.Disp.Z
  Bus Selector4 : BusSelector  OutputSignals=BdyFrm.FrntAxl.Lft.Disp.z,BdyFrm.FrntAxl.Rght.Disp.z,BdyFrm.RearAxl.Lft.Disp.z,BdyFrm.RearAxl.Rght.Disp.z
  Subtract : Sum  Inputs=-+-
  Vector Concatenate{1..4} (4 alike) : Concatenate  NumInputs=4
  Omega : Outport  PortDimensions=4  VectorParamsAs1DForOutWhenUnconnected=off
  Kappa : Outport  Port=2  PortDimensions=4  VectorParamsAs1DForOutWhenUnconnected=off
  Alpha : Outport  Port=3  PortDimensions=4  VectorParamsAs1DForOutWhenUnconnected=off
  XWheel : Outport  Port=4  Unit=m  VectorParamsAs1DForOutWhenUnconnected=off
  YWheel : Outport  Port=5  Unit=m  VectorParamsAs1DForOutWhenUnconnected=off
  ZWheel : Outport  Port=6  PortDimensions=4  VectorParamsAs1DForOutWhenUnconnected=off
  wires:
  Bus Selector1/4 -> Vector Concatenate2/4  "<X>"
  Bus Selector/1 -> Vector Concatenate1/1  "<Y>"
  Bus Selector1/3 -> Vector Concatenate2/3  "<X>"
  Bus Selector/4 -> Vector Concatenate1/4  "<Y>"
  Bus Selector1/2 -> Vector Concatenate2/2  "<X>"
  Bus Selector/3 -> Vector Concatenate1/3  "<Y>"
  Bus Selector/2 -> Vector Concatenate1/2  "<Y>"
  Vector Concatenate1/1 -> YWheel/1
  Bus Selector1/1 -> Vector Concatenate2/1  "<X>"
  Vector Concatenate2/1 -> XWheel/1
  Bus Selector2/1 -> Subtract/3  "<z>"
  Bus Selector2/2 -> Omega/1  "<Omega>"
  Bus Selector2/3 -> Kappa/1  "<Kappa>"
  Bus Selector2/4 -> Alpha/1  "<Alpha>"
  Wheel/1 -> Bus Selector2/1
  Subtract/1 -> ZWheel/1
  Info/1 -> Bus Selector1/1, Bus Selector4/1, Bus Selector3/1, Bus Selector/1
  Bus Selector3/2 -> Vector Concatenate3/2  "<Z>"
  Bus Selector3/3 -> Vector Concatenate3/3  "<Z>"
  Bus Selector3/4 -> Vector Concatenate3/4  "<Z>"
  Bus Selector3/1 -> Vector Concatenate3/1  "<Z>"
  Vector Concatenate3/1 -> Subtract/2
  Vector Concatenate4/1 -> Subtract/1
  Bus Selector4/1 -> Vector Concatenate4/1  "<z>"
  Bus Selector4/4 -> Vector Concatenate4/4  "<z>"
  Bus Selector4/3 -> Vector Concatenate4/3  "<z>"
  Bus Selector4/2 -> Vector Concatenate4/2  "<z>"

== system CAVE_MachE_speedTrack0202/Vehicle Under Test/Vehicle/Vehicle Dynamics/Vehicle 14DOF/Wheels and Tires ==
  Suspension : Inport
  Axle Torque : Inport  Port=2
  Brake Press : Inport  Port=3  Unit=Pa
  Ground Input : Inport  Port=4
  Friction : Inport  Port=5  PortDimensions=4
  Bus Selector1 : BusSelector  OutputSignals=Whl.Ang,Whl.F,Whl.AngVel,Whl.xdot,Whl.ydot
  Constant3 : Constant  Value=zeros(4,1)
  Cont LPF : autolibutils/Cont LPF  wc=100*2*pi  aMode=2
      settings: SourceProductName=Powertrain Blockset  SourceProductBaseCode=PW
  Cont LPF1 : autolibutils/Cont LPF  wc=100*2*pi  aMode=2
      settings: SourceProductName=Powertrain Blockset  SourceProductBaseCode=PW
  Manual Switch6 : ManualSwitch
  Matrix Concatenate : Concatenate  NumInputs=3  Mode=Multidimensional array
  Reshape1 : Reshape
  Reshape2 : Reshape
  Saturation : Saturate  UpperLimit=10*9.81*2040  LowerLimit=-10*9.81*2040  ZeroCross=off
  Selector : Selector  NumberOfDimensions=2  InputPortWidth=3  IndexOptions=Index vector (dialog),Select all  Indices=[3],1  OutputSizes=1,1
  Selector1 : Selector  NumberOfDimensions=2  InputPortWidth=1  IndexOptions=Index vector (dialog),Select all  Indices=[3],1  OutputSizes=1,1
  Selector2 : Selector  NumberOfDimensions=2  InputPortWidth=3  IndexOptions=Index vector (dialog),Select all  Indices=3,1  OutputSizes=1,1
  Selector3 : Selector  NumberOfDimensions=2  InputPortWidth=3  IndexOptions=Index vector (dialog),Select all  Indices=1,1  OutputSizes=1,1
  Terminator{,1,3..5} (5 alike) : Terminator
  VDBS : Subsystem  VariantControl=0
  Wheels : Outport  VectorParamsAs1DForOutWhenUnconnected=off
  wires:
  VDBS/1(Wheels) -> Wheels/1  "Wheels"
  Bus Selector1/2 -> Selector/1  "<F>"
  VDBS/2(FrntAxlF) -> Terminator/1
  VDBS/3(RearAxlF) -> Terminator1/1
  VDBS/4(Omega) -> Terminator3/1
  VDBS/5(Mz) -> Terminator4/1
  Selector1/1 -> Reshape1/1
  Matrix Concatenate/1 -> VDBS/7(VehVel)
  Axle Torque/1 -> VDBS/3(AxleTrq)
  Selector2/1 -> VDBS/1(WheelAng)  "Wheel Angles"
  Constant3/1 -> Manual Switch6/1
  Manual Switch6/1 -> VDBS/2(CamberAng)  "Camber Angles"
  Selector/1 -> Reshape2/1
  Saturation/1 -> VDBS/5(Fz)
  Ground Input/1 -> VDBS/8(Ground Level)
  VDBS/7(SuspWhlVz) -> Matrix Concatenate/3  "zdot"
  Bus Selector1/1 -> Cont LPF1/1  "<Ang>"
  Selector3/1 -> Manual Switch6/2  "Camber Angles"
  Suspension/1 -> Bus Selector1/1
  Bus Selector1/4 -> Matrix Concatenate/1  "<xdot>"
  Bus Selector1/5 -> Matrix Concatenate/2  "<ydot>"
  VDBS/6(SuspWhlPz) -> Terminator5/1  "z"
  Reshape2/1 -> Cont LPF/1
  Bus Selector1/3 -> Selector1/1  "<AngVel>"
  Reshape1/1 -> VDBS/6(r)
  Brake Press/1 -> VDBS/4(BrkPrs)
  Friction/1 -> VDBS/9(Friction)
  Cont LPF/1 -> Saturation/1
  Cont LPF1/1 -> Selector3/1, Selector2/1

== system CAVE_MachE_speedTrack0202/Vehicle Under Test/Vehicle/Vehicle Dynamics/Vehicle 7DOF/Brake Pressure ==
  BrkReq : Inport
  Bus Creator1 : BusCreator  Inputs=2
  Gain : Gain  Gain=BrakeMaxPrs
  Gain{1..4} (4 alike) : Gain  Gain=0.5
  Saturation{,1..3} (4 alike) : Saturate  UpperLimit=BrakeMaxPrs  LowerLimit=0  ZeroCross=off
  Signal Specification : SignalSpecification  Unit=Pa
  Terminator : Terminator
  Vector Concatenate2 : Concatenate  NumInputs=4
  BrakePrs : Outport  Unit=Pa
  wires:
  BrkReq/1 -> Gain/1, Bus Creator1/1  "BrkReq"
  Gain/1 -> Signal Specification/1
  Signal Specification/1 -> Gain2/1, Gain1/1, Bus Creator1/2  "BrkPrs"
  Bus Creator1/1 -> Terminator/1  "WhlBrk"
  Gain1/1 -> Gain4/1
  Gain2/1 -> Gain3/1
  Gain3/1 -> Saturation/1, Saturation1/1
  Gain4/1 -> Saturation2/1, Saturation3/1
  Vector Concatenate2/1 -> BrakePrs/1
  Saturation/1 -> Vector Concatenate2/1
  Saturation1/1 -> Vector Concatenate2/2
  Saturation2/1 -> Vector Concatenate2/3
  Saturation3/1 -> Vector Concatenate2/4

== system CAVE_MachE_speedTrack0202/Vehicle Under Test/Vehicle/Vehicle Dynamics/Vehicle 7DOF/Longitudinal Wheels 4DOF ==
  WhlAng : Inport
  AxlTrq : Inport  Port=2
  BrkPrs : Inport  Port=3
  Gnd : Inport  Port=4  PortDimensions=4
  lam_mu : Inport  Port=5  PortDimensions=4
  VehFdbk : Inport  Port=6
  Axle Forces : Subsystem  VariantControlMode=Label  Variant=on  LabelModeActiveChoice=1
  Bus Selector5 : BusSelector  OutputSignals=BdyFrm.Cg.AngVel.r
  Constant : vehdynlibtirecommon/Constant  const=220000  numWheels=4
      settings: SourceProductName=Vehicle Dynamics Blockset  SourceProductBaseCode=VE
  Constant3 : vehdynlibtirecommon/Constant  const=0  numWheels=4
      settings: SourceProductName=Vehicle Dynamics Blockset  SourceProductBaseCode=VE
  Terminator2 : Terminator
  Tire2Veh : Subsystem
  Tires : Subsystem
  Veh2Tire : Subsystem
  Velocity and Vertical Load : Subsystem  VariantControlMode=Label  Variant=on  LabelModeActiveChoice=1
  Wheel Angles : Subsystem
  FrntAxlF : Outport  Unit=N  VectorParamsAs1DForOutWhenUnconnected=off
  RearAxlF : Outport  Port=2  Unit=N  VectorParamsAs1DForOutWhenUnconnected=off
  Omega : Outport  Port=3  VectorParamsAs1DForOutWhenUnconnected=off
  Kappa : Outport  Port=4  VectorParamsAs1DForOutWhenUnconnected=off
  Alpha : Outport  Port=5  VectorParamsAs1DForOutWhenUnconnected=off
  zAxle : Outport  Port=6  VectorParamsAs1DForOutWhenUnconnected=off
  wires:
  Wheel Angles/1(WhlAngB) -> Veh2Tire/5(WhlAng)
  Tires/1(Wheel) -> Tire2Veh/1(Wheel)
  lam_mu/1 -> Tires/9(lam_mu)
  Constant/1 -> Tires/7(TirePrs)
  Constant3/1 -> Wheel Angles/2(Camber), Tires/6(Camber)
  Veh2Tire/3(xdotAxle) -> Tires/3(Vx)  "Vx"
  Gnd/1 -> Tires/10(Gnd)
  VehFdbk/1 -> Bus Selector5/1, Velocity and Vertical Load/1(VehFdbk)
  AxlTrq/1 -> Veh2Tire/1(AxlTrq)
  Veh2Tire/1(T) -> Tires/1(AxlTrq)
  Veh2Tire/2(P) -> Tires/2(BrkPrs)
  BrkPrs/1 -> Veh2Tire/2(BrkPrs)
  Bus Selector5/1 -> Veh2Tire/3(r)  "<r>"
  Veh2Tire/6(zdotAxle) -> Terminator2/1
  WhlAng/1 -> Wheel Angles/1(WheelAng)  "FrontWheelAngles"
  Veh2Tire/4(ydotAxle) -> Tires/4(Vy)  "Vy"
  Veh2Tire/5(psidot) -> Tires/5(r)
  Velocity and Vertical Load/2(Fz) -> Tires/8(Fz)
  Velocity and Vertical Load/1(VehVel) -> Veh2Tire/4(VehVel)
  Axle Forces/1(FrntAxlF) -> FrntAxlF/1
  Axle Forces/2(RearAxlF) -> RearAxlF/1
  Tire2Veh/1(FwF) -> Axle Forces/1(F)
  Tire2Veh/2(FwR) -> Axle Forces/2(R)
  Tire2Veh/3(z) -> zAxle/1
  Tire2Veh/4(Omega) -> Omega/1
  Tire2Veh/5(Kappa) -> Kappa/1
  Tire2Veh/6(Alpha) -> Alpha/1

== system CAVE_MachE_speedTrack0202/Vehicle Under Test/Vehicle/Vehicle Dynamics/Vehicle 7DOF/RototestDummy ==
  Bus Creator1 : BusCreator  Inputs=ActTqLF_Nm_,ActTqRF_Nm_,ActTqLR_Nm_,ActTqRR_Nm_
  Bus Creator2 : BusCreator  Inputs=Car Trq_T2WFL,Car Trq_T2WFR,Car Trq_T2WRL,Car Trq_T2WRR
  Bus Creator3 : BusCreator  Inputs=1
  Bus Creator4 : BusCreator  Inputs=1
  Bus Selector14 : BusSelector  OutputSignals=VehSpd
  Bus Selector15 : BusSelector  OutputSignals=TireFrame.Fx
  Constant{1..14} (14 alike) : Constant  Value=0
  Vector Concatenate3 : Concatenate  NumInputs=4
  CarTrqT2W : Outport
  AxleTrq : Outport  Port=2
  BrakePressed_flag : Outport  Port=3
  <VehSpd> : Outport  Port=4
  <Fx> : Outport  Port=5
  wires:
  Constant10/1 -> Bus Selector14/1  "VehSpd"
  Bus Creator4/1 -> Bus Creator3/1  "TireFrame"
  Bus Creator1/1 -> AxleTrq/1  "AxleTrq"
  Constant9/1 -> Bus Creator1/4  "ActTqRR_Nm_"
  Constant13/1 -> Bus Creator2/3  "CarTrq_T2WRL"
  Constant4/1 -> Vector Concatenate3/4
  Bus Creator3/1 -> Bus Selector15/1
  Vector Concatenate3/1 -> Bus Creator4/1  "Fx"
  Constant3/1 -> Vector Concatenate3/3
  Constant2/1 -> Vector Concatenate3/2
  Constant14/1 -> Bus Creator2/4  "CarTrq_T2WRR"
  Constant6/1 -> Bus Creator1/1  "ActTqLF_Nm_"
  Constant1/1 -> Vector Concatenate3/1
  Constant8/1 -> Bus Creator1/3  "ActTqLR_Nm_"
  Constant11/1 -> Bus Creator2/1  "CarTrq_T2WFL"
  Constant7/1 -> Bus Creator1/2  "ActTqRF_Nm_"
  Constant12/1 -> Bus Creator2/2  "CarTrq_T2WFR"
  Bus Creator2/1 -> CarTrqT2W/1  "CarTrqT2W"
  Bus Selector14/1 -> <VehSpd>/1  "<VehSpd>"
  Constant5/1 -> BrakePressed_flag/1  "BrakePressed_flag"
  Bus Selector15/1 -> <Fx>/1  "<Fx>"

== system CAVE_MachE_speedTrack0202/Vehicle Under Test/Vehicle/Vehicle Dynamics/Vehicle 7DOF/Steering ==
  SteeringCmd : Inport
  Ground : Ground
  Kinematic Steering : vehdynlibsteering/Kinematic Steering  StrgType=Ackerman  StrgRatioType=Constant  Loc=Front  NrmlFctr=1  TrckWdth=1.9  WhlBase=ChassisDistCg2FrontAxle+ChassisDistCg2RearAxle  Db=0  StrgRng=3*pi  StrgAngBpts="[-6.2832   -5.0265   -3.7699   -2.5133   -1.2566         0    1.2566    2.5133    3.7699    5.0265    6.2832]"  StrgRatioTbl=|  StrgRatio=18  StrgArmLngth=0.1  RckCsLngth=0.5  TieRodLngth=0.248  D=0.2  PnnRadius=0.0057  PnnRadiusTbl="[0.0055    0.0055    0.0056    0.0057    0.0058    0.0057    0.0057    0.0057    0.0056    0.0055    0.0055]"  RodLngth=0.1  ParaArmLngth=0.9  aMode=2
      | [13.5000   13.3750   13.2500   13.1250   13.0000   13.0000   13.0000   13.1250   13.2500   13.3750   13.5000
      | ]
      settings: SourceProductName=Vehicle Dynamics Blockset
  Terminator1 : Terminator
  Vector Concatenate : Concatenate
  Vector Concatenate1 : Concatenate
  Vector Concatenate2 : Concatenate
  WhlAng : Outport  Unit=rad
  wires:
  Kinematic Steering/1 -> Terminator1/1
  Vector Concatenate2/1 -> WhlAng/1
  Kinematic Steering/2 -> Vector Concatenate/1
  Vector Concatenate1/1 -> Vector Concatenate2/2  "RearWheelAngles"
  Vector Concatenate/1 -> Vector Concatenate2/1  "FrontWheelAngles"
  Ground/1 -> Vector Concatenate1/2, Vector Concatenate1/1
  Kinematic Steering/3 -> Vector Concatenate/2
  SteeringCmd/1 -> Kinematic Steering/1
